simulink model "input_shaping"  (R2025b)
settings: Solver=VariableStepAuto  StartTime=0.0  StopTime=20  RelTol=1e-3
libraries: simulink x4
settings Model: Creator=David  LastModifiedBy=David

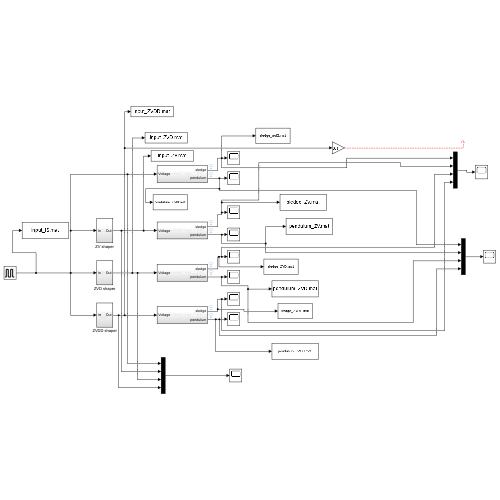
[thumbnail: Simulink's stored preview of the top-level diagram]
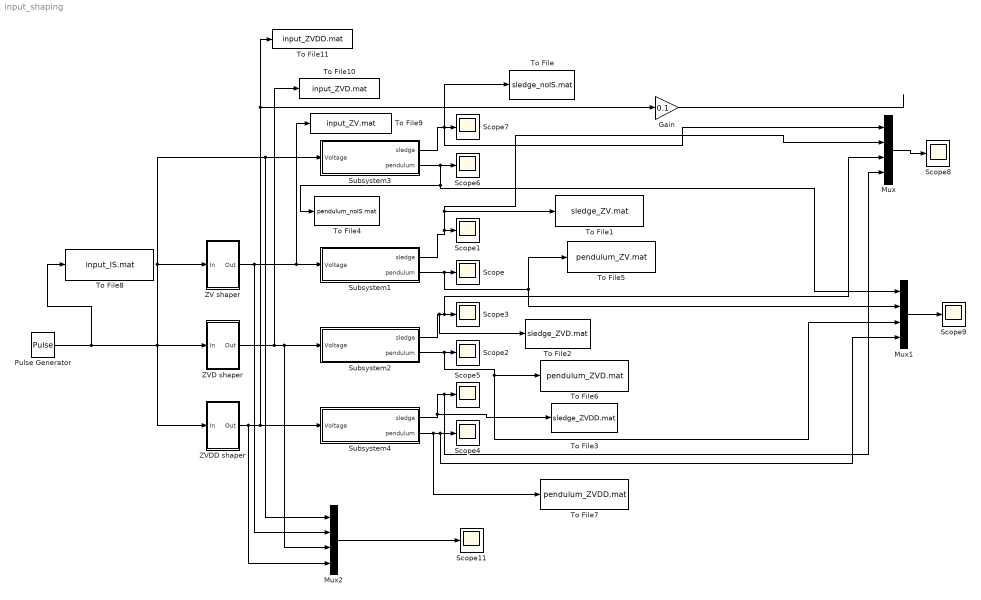
== system input_shaping ==
  Gain : Gain  Gain=0.1
  Mux : Mux
  Mux1 : Mux
  Mux2 : Mux
  Pulse Generator : DiscretePulseGenerator  PulseType=Time based  Amplitude=4  Period=50  PulseWidth=5  PhaseDelay=2
  Scope{,1..9,11} (11 alike) : Scope
      Scope settings: ActiveDisplayYMinimum=-1  ActiveDisplayYMaximum=1
      Scope1 settings: ActiveDisplayYMinimum=-1  ActiveDisplayYMaximum=1  DataLoggingVariableName=ScopeData3
      Scope11 settings: ActiveDisplayYMinimum=-1  ActiveDisplayYMaximum=1  DataLoggingVariableName=ScopeData14
      Scope2 settings: ActiveDisplayYMinimum=-0.16064529340853845  ActiveDisplayYMaximum=0.1569195069828942  DataLoggingVariableName=ScopeData4
      Scope3 settings: ActiveDisplayYMinimum=-1  ActiveDisplayYMaximum=1  DataLoggingVariableName=ScopeData5
      Scope4 settings: ActiveDisplayYMinimum=-1  ActiveDisplayYMaximum=1  DataLoggingVariableName=ScopeData6
      Scope5 settings: ActiveDisplayYMinimum=-1  ActiveDisplayYMaximum=1  DataLoggingVariableName=ScopeData7
      Scope6 settings: ActiveDisplayYMinimum=-1  ActiveDisplayYMaximum=1  DataLoggingVariableName=ScopeData8
      Scope7 settings: ActiveDisplayYMinimum=-1  ActiveDisplayYMaximum=1  DataLoggingVariableName=ScopeData9
      Scope8 settings: ActiveDisplayYMinimum=-0.063491061508938421  ActiveDisplayYMaximum=0.57141955358044594  DataLoggingVariableName=ScopeData11
      Scope9 settings: ActiveDisplayYMinimum=-0.24624561695994068  ActiveDisplayYMaximum=0.24088756642140846  DataLoggingVariableName=ScopeData12
  Subsystem1 : Subsystem
  Subsystem2 : Subsystem
  Subsystem3 : Subsystem
  Subsystem4 : Subsystem
  To File : ToFile  Filename=sledge_noIS.mat  SaveFormat=Timeseries
  To File1 : ToFile  Filename=sledge_ZV.mat  SaveFormat=Timeseries
  To File10 : ToFile  Filename=input_ZVD.mat  SaveFormat=Timeseries
  To File11 : ToFile  Filename=input_ZVDD.mat  SaveFormat=Timeseries
  To File2 : ToFile  Filename=sledge_ZVD.mat  SaveFormat=Timeseries
  To File3 : ToFile  Filename=sledge_ZVDD.mat  SaveFormat=Timeseries
  To File4 : ToFile  Filename=pendulum_noIS.mat  SaveFormat=Timeseries
  To File5 : ToFile  Filename=pendulum_ZV.mat  SaveFormat=Timeseries
  To File6 : ToFile  Filename=pendulum_ZVD.mat  SaveFormat=Timeseries
  To File7 : ToFile  Filename=pendulum_ZVDD.mat  SaveFormat=Timeseries
  To File8 : ToFile  Filename=input_IS.mat  SaveFormat=Timeseries
  To File9 : ToFile  Filename=input_ZV.mat  SaveFormat=Timeseries
  ZV shaper : Subsystem
  ZVD shaper : Subsystem
  ZVDD shaper : Subsystem
  wires:
  Pulse Generator/1 -> To File8/1, ZVDD shaper/1(In), Subsystem3/1(Voltage), Mux2/1, ZV shaper/1(In), ZVD shaper/1(In)
  ZV shaper/1(Out) -> Mux2/2, Subsystem1/1(Voltage), To File9/1
  Subsystem1/2(pendulum) -> To File5/1, Mux1/2, Scope/1
  Subsystem1/1(sledge) -> Mux/2, To File1/1, Scope1/1
  Subsystem2/1(sledge) -> To File2/1, Mux/3, Scope3/1
  Subsystem2/2(pendulum) -> Mux1/3, To File6/1, Scope2/1
  Subsystem4/1(sledge) -> Mux/4, Scope5/1, To File3/1
  Subsystem4/2(pendulum) -> To File7/1, Mux1/4, Scope4/1
  ZVDD shaper/1(Out) -> Mux2/4, Subsystem4/1(Voltage), To File11/1, Gain/1
  ZVD shaper/1(Out) -> To File10/1, Subsystem2/1(Voltage), Mux2/3
  Subsystem3/1(sledge) -> To File/1, Mux/1, Scope7/1
  Subsystem3/2(pendulum) -> Mux1/1, To File4/1, Scope6/1
  Mux1/1 -> Scope9/1
  Mux/1 -> Scope8/1
  Mux2/1 -> Scope11/1
  Gain/1 -> ?

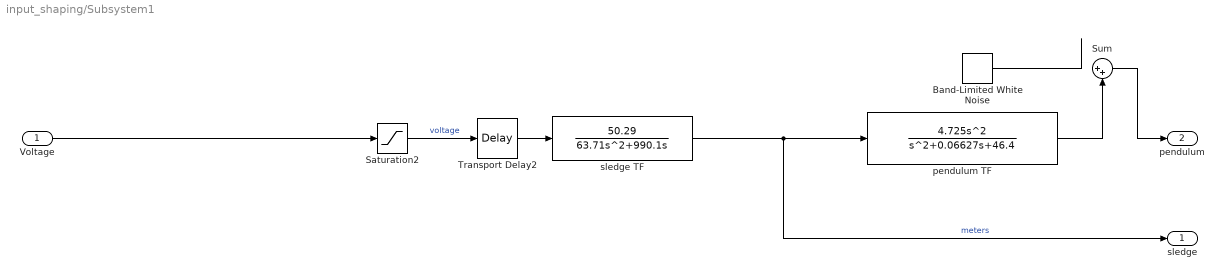
== system input_shaping/Subsystem1 ==
  Voltage : Inport
  Band-Limited White Noise : simulink/Sources/Band-Limited White Noise  Cov=[4.9008e-09]  Ts=0.01  seed=[23341]
  Saturation2 : Saturate  UpperLimit=12  LowerLimit=-12
  Sum : Sum  Inputs=|++
  Transport Delay2 : TransportDelay  DelayTime=0.01
  pendulum TF : TransferFcn  Numerator=[4.725 0 0]  Denominator=[1 0.06627 46.4]
  sledge TF : TransferFcn  Numerator=50.29  Denominator="[63.71  990.1 0]"
  sledge : Outport
  pendulum : Outport  Port=2
  wires:
  Saturation2/1 -> Transport Delay2/1  "voltage"
  sledge TF/1 -> pendulum TF/1, sledge/1  "meters"
  pendulum TF/1 -> Sum/2
  Band-Limited White Noise/1 -> ?
  Sum/1 -> pendulum/1
  Voltage/1 -> Saturation2/1
  Transport Delay2/1 -> sledge TF/1

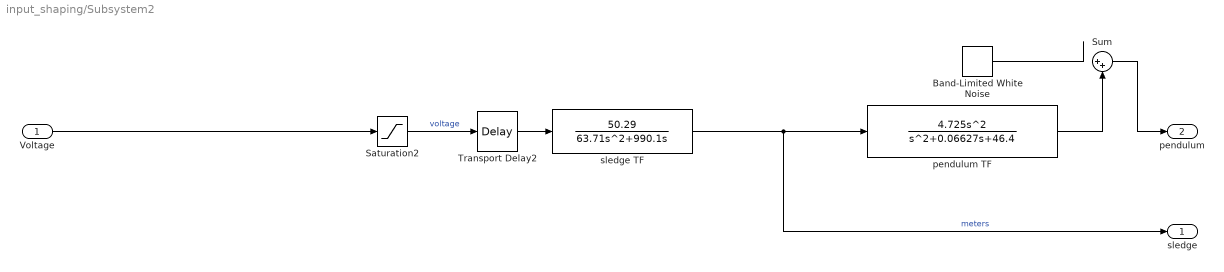
== system input_shaping/Subsystem2 ==
  Voltage : Inport
  Band-Limited White Noise : simulink/Sources/Band-Limited White Noise  Cov=[4.9008e-09]  Ts=0.01  seed=[23341]
  Saturation2 : Saturate  UpperLimit=12  LowerLimit=-12
  Sum : Sum  Inputs=|++
  Transport Delay2 : TransportDelay  DelayTime=0.01
  pendulum TF : TransferFcn  Numerator=[4.725 0 0]  Denominator=[1 0.06627 46.4]
  sledge TF : TransferFcn  Numerator=50.29  Denominator="[63.71  990.1 0]"
  sledge : Outport
  pendulum : Outport  Port=2
  wires:
  Saturation2/1 -> Transport Delay2/1  "voltage"
  sledge TF/1 -> pendulum TF/1, sledge/1  "meters"
  pendulum TF/1 -> Sum/2
  Band-Limited White Noise/1 -> ?
  Sum/1 -> pendulum/1
  Voltage/1 -> Saturation2/1
  Transport Delay2/1 -> sledge TF/1

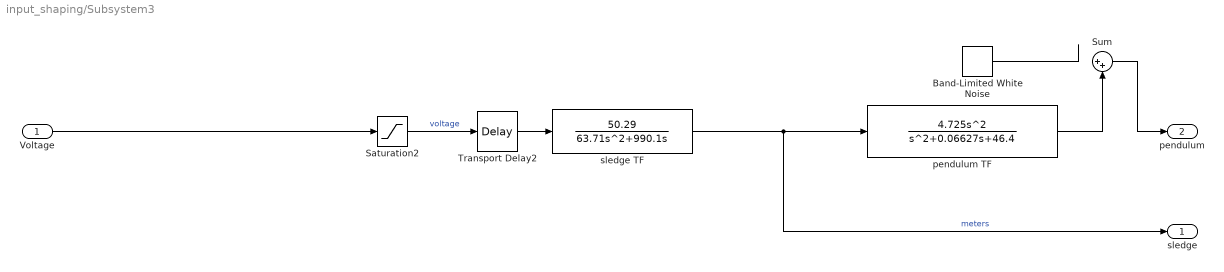
== system input_shaping/Subsystem3 ==
  Voltage : Inport
  Band-Limited White Noise : simulink/Sources/Band-Limited White Noise  Cov=[4.9008e-09]  Ts=0.01  seed=[23341]
  Saturation2 : Saturate  UpperLimit=12  LowerLimit=-12
  Sum : Sum  Inputs=|++
  Transport Delay2 : TransportDelay  DelayTime=0.01
  pendulum TF : TransferFcn  Numerator=[4.725 0 0]  Denominator=[1 0.06627 46.4]
  sledge TF : TransferFcn  Numerator=50.29  Denominator="[63.71  990.1 0]"
  sledge : Outport
  pendulum : Outport  Port=2
  wires:
  Saturation2/1 -> Transport Delay2/1  "voltage"
  sledge TF/1 -> pendulum TF/1, sledge/1  "meters"
  pendulum TF/1 -> Sum/2
  Band-Limited White Noise/1 -> ?
  Sum/1 -> pendulum/1
  Voltage/1 -> Saturation2/1
  Transport Delay2/1 -> sledge TF/1

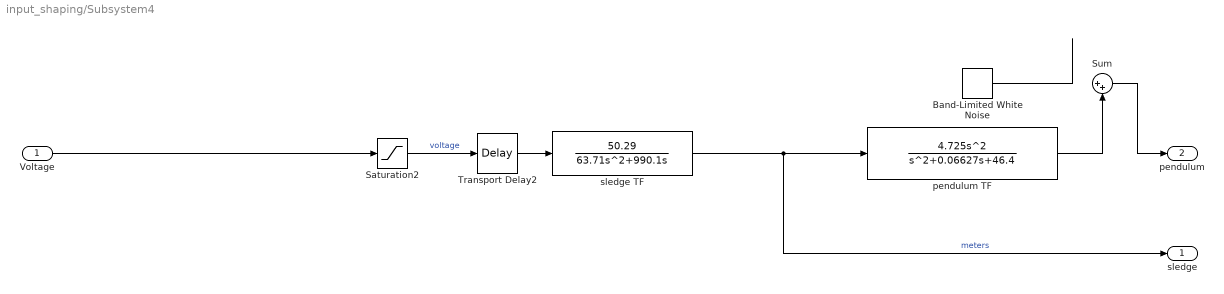
== system input_shaping/Subsystem4 ==
  Voltage : Inport
  Band-Limited White Noise : simulink/Sources/Band-Limited White Noise  Cov=[4.9008e-09]  Ts=0.01  seed=[23341]
  Saturation2 : Saturate  UpperLimit=12  LowerLimit=-12
  Sum : Sum  Inputs=|++
  Transport Delay2 : TransportDelay  DelayTime=0.01
  pendulum TF : TransferFcn  Numerator=[4.725 0 0]  Denominator=[1 0.06627 46.4]
  sledge TF : TransferFcn  Numerator=50.29  Denominator="[63.71  990.1 0]"
  sledge : Outport
  pendulum : Outport  Port=2
  wires:
  Saturation2/1 -> Transport Delay2/1  "voltage"
  sledge TF/1 -> pendulum TF/1, sledge/1  "meters"
  pendulum TF/1 -> Sum/2
  Band-Limited White Noise/1 -> ?
  Sum/1 -> pendulum/1
  Voltage/1 -> Saturation2/1
  Transport Delay2/1 -> sledge TF/1

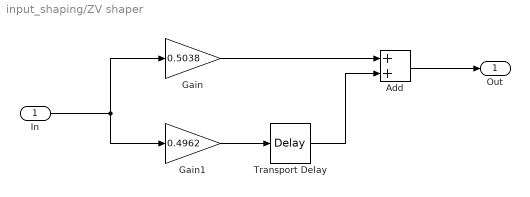
== system input_shaping/ZV shaper ==
  In : Inport
  Add : Sum
  Gain : Gain  Gain=0.5038
  Gain1 : Gain  Gain=0.4962
  Transport Delay : TransportDelay  DelayTime=0.4612
  Out : Outport
  wires:
  Add/1 -> Out/1
  In/1 -> Gain/1, Gain1/1
  Gain1/1 -> Transport Delay/1
  Transport Delay/1 -> Add/2
  Gain/1 -> Add/1

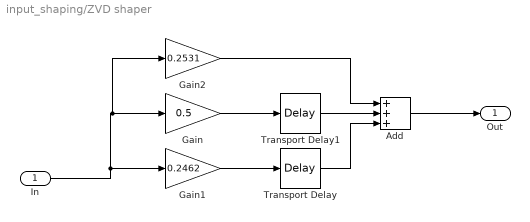
== system input_shaping/ZVD shaper ==
  In : Inport
  Add : Sum  Inputs=+++
  Gain : Gain  Gain=0.5
  Gain1 : Gain  Gain=0.2462
  Gain2 : Gain  Gain=0.2531
  Transport Delay : TransportDelay  DelayTime=0.9224
  Transport Delay1 : TransportDelay  DelayTime=0.4607
  Out : Outport
  wires:
  Gain/1 -> Transport Delay1/1
  Gain1/1 -> Transport Delay/1
  In/1 -> Gain1/1, Gain2/1, Gain/1
  Add/1 -> Out/1
  Transport Delay1/1 -> Add/2
  Transport Delay/1 -> Add/3
  Gain2/1 -> Add/1

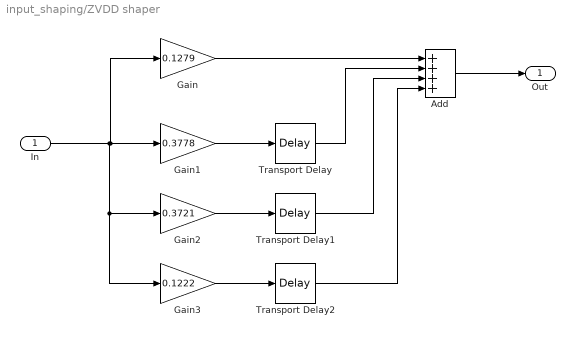
== system input_shaping/ZVDD shaper ==
  In : Inport
  Add : Sum  Inputs=++++
  Gain : Gain  Gain=0.1279
  Gain1 : Gain  Gain=0.3778
  Gain2 : Gain  Gain=0.3721
  Gain3 : Gain  Gain=0.1222
  Transport Delay : TransportDelay  DelayTime=0.4612
  Transport Delay1 : TransportDelay  DelayTime=0.9224
  Transport Delay2 : TransportDelay  DelayTime=1.3836
  Out : Outport
  wires:
  Add/1 -> Out/1
  In/1 -> Gain/1, Gain1/1, Gain3/1, Gain2/1
  Gain1/1 -> Transport Delay/1
  Transport Delay/1 -> Add/2
  Gain/1 -> Add/1
  Gain3/1 -> Transport Delay2/1
  Gain2/1 -> Transport Delay1/1
  Transport Delay1/1 -> Add/3
  Transport Delay2/1 -> Add/4
